simulink model "nuclear"  (Simulink 7.8)
settings: Solver=ode45  StartTime=0.0  StopTime=24  RelTol=1e-3
libraries: simulink x1
settings Model: Creator=John  LastModifiedBy=John
settings DebuggingCC: SolverPrmCheckMsg=none

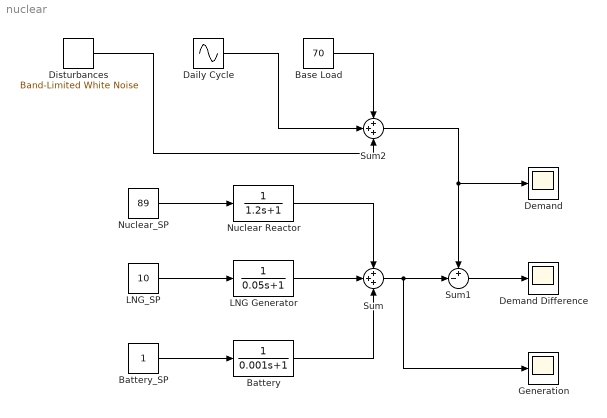
== system nuclear ==
  Base Load : Constant  Value=70
  Battery : TransferFcn  Denominator=[0.001 1]
  Battery_SP : Constant
  Daily Cycle : Sin  Amplitude=20  Frequency=2*3.1415/24  SampleTime=0
  Demand : Scope
  Demand Difference : Scope
  Disturbances : simulink/Sources/Band-Limited White Noise  Cov=[5]  Ts=0.5  seed=[23342]
  Generation : Scope
      settings: SaveName=ScopeData2
  LNG Generator : TransferFcn  Denominator=[0.05 1]
  LNG_SP : Constant  Value=10
  Nuclear Reactor : TransferFcn  Denominator=[1.2 1]
  Nuclear_SP : Constant  Value=89
  Sum : Sum  Inputs=+++
  Sum1 : Sum  Inputs=+-|
  Sum2 : Sum  Inputs=+++
  wires:
  Nuclear_SP/1 -> Nuclear Reactor/1
  Nuclear Reactor/1 -> Sum/1
  LNG_SP/1 -> LNG Generator/1
  LNG Generator/1 -> Sum/2
  Battery_SP/1 -> Battery/1
  Battery/1 -> Sum/3
  Sum/1 -> Sum1/2, Generation/1
  Sum1/1 -> Demand Difference/1
  Base Load/1 -> Sum2/1
  Daily Cycle/1 -> Sum2/2
  Disturbances/1 -> Sum2/3
  Sum2/1 -> Sum1/1, Demand/1
